simulink model "pendulum_func"  (R2019b)
settings: Solver=VariableStepAuto  StartTime=0.0  StopTime=10.0  RelTol=1e-3
settings Model: Creator=Admin  LastModifiedBy=Admin

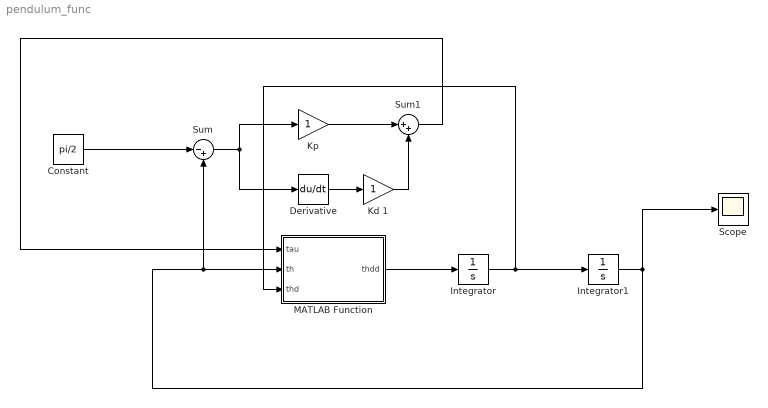
== system pendulum_func ==
  Constant : Constant  Value=pi/2
  Derivative : Derivative
  Integrator : Integrator
  Integrator1 : Integrator
  Kd 1 : Gain
  "Kp " : Gain
  MATLAB Function : MATLAB Function  TreatAsAtomicUnit=on
  Scope : Scope
  Sum : Sum  Inputs=|-+
  Sum1 : Sum  Inputs=|++
  wires:
  MATLAB Function/1(thdd) -> Integrator/1
  Integrator/1 -> MATLAB Function/3(thd), Integrator1/1
  Integrator1/1 -> Scope/1, MATLAB Function/2(th), Sum/2
  Constant/1 -> Sum/1
  Sum/1 -> "Kp "/1, Derivative/1
  "Kp "/1 -> Sum1/1
  Sum1/1 -> MATLAB Function/1(tau)
  Derivative/1 -> Kd 1/1
  Kd 1/1 -> Sum1/2

== matlab function pendulum_func/MATLAB Function ==
  data: tau input; thdd output; th input; thd input
function thdd = Pendulum(tau,th,thd)
m=1;
g=9.8;
l=1;

thdd = (-tau+m*g*l*sin(th))/(m*l^2)-0.5*thd;
end
